simulink model "Sliding_Mode_Slotine_Regressor"  (R2018b)
settings: Solver=FixedStepAuto  StartTime=0.0  StopTime=10  FixedStep=0.001  RelTol=1e-3
values from neighbouring files (symbols this model uses):
  F1G = 0.2    [Main_Code.m]    (also in Main_Code_Gravity_Compensation.m)
  F2G = 0.2    [Main_Code.m]    (also in Main_Code_Gravity_Compensation.m)
  F3G = 0.005    [Main_Code.m]    (also in Main_Code_Gravity_Compensation.m)
  Gauss_B = [0 0 0 0 0 0 0 0 0 0 0 0 ... (1200 elements, 15x80)]    [Gauss_Jordan.mat]
  Gauss_BB = [0 0 0 0 0 0 0 0 0 0 0 0 ... (1200 elements, 80x15)]    [Gauss_Jordan.mat]
  phi_Dynamic = [phi0;phi1;phi2;phi3;phi4;phi5;phi6;phi7]    [Parameters_Builder.m]    (also in Robot_Parameters.mat = [0.73163251 -0.0393 0 2.40643096032e-18 0.000785329049449 0.; Robot_Parameters_Ident.mat = [0.78122 -0.0393 0 2.40643096032e-18 0.000785329049449 0.000; Robot_Parameters_Ident_With_Disturbance.mat = [0.78122 -0.0393 0 2.40643096032e-18 0.000785329049449 0.000)
  phi_Kinematic = [l__0;l__1;l__3;l__5;l__2;l__7;theta;alpha;d__0;l__x35;l__z35;psi0]    [Parameters_Builder.m]    (also in Robot_Parameters.mat = [0.006 0.182 0.05 0.115 0.07 0.0342 0.733038285838 0.8726646; Robot_Parameters_Ident.mat = [0.006 0.182 0.05 0.115 0.07 0.0342 0.733038285838 0.8726646; Robot_Parameters_Ident_With_Disturbance.mat = [0.006 0.182 0.05 0.115 0.07 0.0342 0.733038285838 0.8726646)
undefined symbols (not defined in the file or in its folder): gamma, K
libraries: slrtlib x5, xpcrtudplib x3, xpcutilitieslib x2
settings Model: Creator=Legend  LastModifiedBy=ARAS
settings SFSimCC: SimUseLocalCustomCode=off
settings RTWCC: RTWUseLocalCustomCode=off
settings CodeAppCC: StateflowObjectComments=on

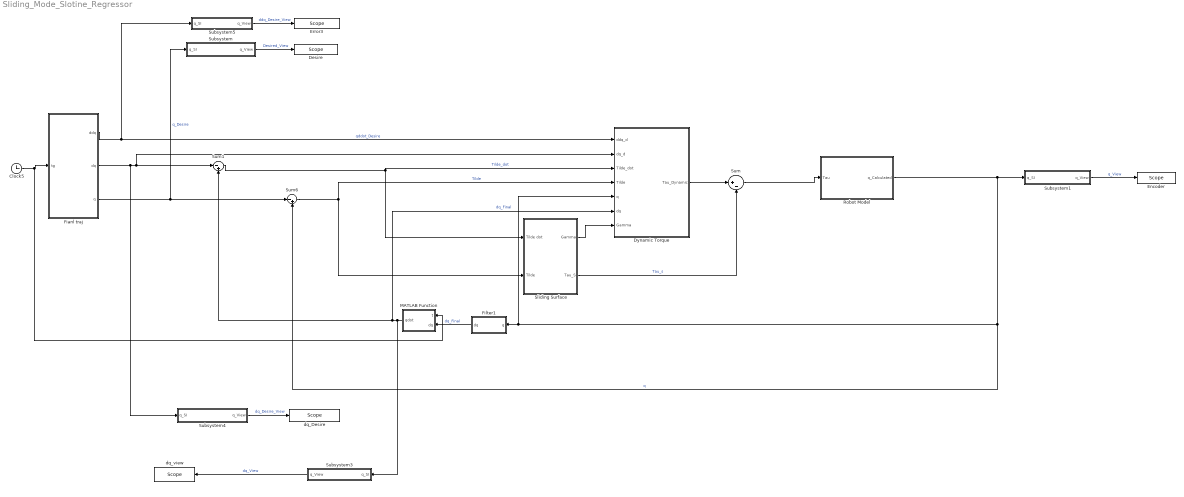
== system Sliding_Mode_Slotine_Regressor ==
  Clock5 : Clock
  Desire : slrtlib/Displays and Logging/Scope   scopeno=2  scopetype=Target  autostart=on  viewmode=Numerical  formatstr='%15.6f'  grid=on  ylimits=[0,0]  nosamples=3  noprepostsamples=0  interleave=1  triggermode=FreeRun  triggersignal=1  trigsignalfromport=off  triggerlevel=0.0  triggerslope=Either  triggerscope=1  triggersample=0  filename=data.dat  mode=Lazy  writesize=512  autorestart=off  dynamicfilemode=off  maxwritefilesize=512*1024^2
  Dynamic Torque : Subsystem
  Encoder : slrtlib/Displays and Logging/Scope   scopeno=1  scopetype=Target  autostart=on  viewmode=Numerical  formatstr='%15.6f'  grid=on  ylimits=[0,0]  nosamples=3  noprepostsamples=0  interleave=1  triggermode=FreeRun  triggersignal=1  trigsignalfromport=off  triggerlevel=0.0  triggerslope=Either  triggerscope=1  triggersample=0  filename=data.dat  mode=Lazy  writesize=512  autorestart=off  dynamicfilemode=off  maxwritefilesize=512*1024^2
  Error3 : slrtlib/Displays and Logging/Scope   scopeno=3  scopetype=Target  autostart=on  viewmode=Numerical  formatstr='%15.6f'  grid=on  ylimits=[0,0]  nosamples=3  noprepostsamples=0  interleave=1  triggermode=FreeRun  triggersignal=1  trigsignalfromport=off  triggerlevel=0.0  triggerslope=Either  triggerscope=1  triggersample=0  filename=data.dat  mode=Lazy  writesize=512  autorestart=off  dynamicfilemode=off  maxwritefilesize=512*1024^2
  Fianl traj : MATLAB Function  TreatAsAtomicUnit=on
  Filter1 : Subsystem
  MATLAB Function : MATLAB Function  TreatAsAtomicUnit=on
  Robot Model : Subsystem
  Sliding Surface : Subsystem
  Subsystem : Subsystem
  Subsystem1 : Subsystem
  Subsystem3 : Subsystem
  Subsystem4 : Subsystem
  Subsystem5 : Subsystem
  Sum : Sum  Inputs=|+-
  Sum1 : Sum  Inputs=|-+
  Sum6 : Sum  Inputs=|-+
  dq_Desire : slrtlib/Displays and Logging/Scope   scopeno=4  scopetype=Target  autostart=on  viewmode=Numerical  formatstr='%15.6f'  grid=on  ylimits=[0,0]  nosamples=3  noprepostsamples=0  interleave=1  triggermode=FreeRun  triggersignal=1  trigsignalfromport=off  triggerlevel=0.0  triggerslope=Either  triggerscope=1  triggersample=0  filename=data.dat  mode=Lazy  writesize=512  autorestart=off  dynamicfilemode=off  maxwritefilesize=512*1024^2
  dq_view : slrtlib/Displays and Logging/Scope   scopeno=5  scopetype=Target  autostart=on  viewmode=Numerical  formatstr='%15.6f'  grid=on  ylimits=[0,0]  nosamples=3  noprepostsamples=0  interleave=1  triggermode=FreeRun  triggersignal=1  trigsignalfromport=off  triggerlevel=0.0  triggerslope=Either  triggerscope=1  triggersample=0  filename=data.dat  mode=Lazy  writesize=512  autorestart=off  dynamicfilemode=off  maxwritefilesize=512*1024^2
  wires:
  MATLAB Function/1(qdot) -> Sum1/2, Dynamic Torque/6(dq), Subsystem3/1(q_SI)  "dq_Final"
  Robot Model/1(q_Calculated) -> Subsystem1/1(q_SI), Dynamic Torque/5(q), Filter1/1(q), Sum6/2  "q"
  Clock5/1 -> MATLAB Function/1(t), Fianl traj/1(tg)
  Sum6/1 -> Dynamic Torque/4(Tilde), Sliding Surface/2(Tilde)  "Tilde"
  Sum1/1 -> Sliding Surface/1(Tilde dot), Dynamic Torque/3(Tilde_dot)  "Tilde_dot"
  Fianl traj/1(ddq) -> Subsystem5/1(q_SI), Dynamic Torque/1(ddq_d)  "qddot_Desire"
  Sum/1 -> Robot Model/1(Tau)
  Dynamic Torque/1(Tau_Dynamic) -> Sum/1
  Sliding Surface/2(Tau_S) -> Sum/2  "Tau_s"
  Sliding Surface/1(Gamma) -> Dynamic Torque/7(Gamma)
  Subsystem1/1(q_View) -> Encoder/1  "q_View"
  Fianl traj/3(q) -> Subsystem/1(q_SI), Sum6/1  "q_Desire"
  Fianl traj/2(dq) -> Dynamic Torque/2(dq_d), Sum1/1, Subsystem4/1(q_SI)
  Subsystem5/1(q_View) -> Error3/1  "ddq_Desire_View"
  Subsystem/1(q_View) -> Desire/1  "Desired_View"
  Subsystem4/1(q_View) -> dq_Desire/1  "dq_Desire_View"
  Filter1/1(dq) -> MATLAB Function/2(dq)  "dq_Final"
  Subsystem3/1(q_View) -> dq_view/1  "dq_View"

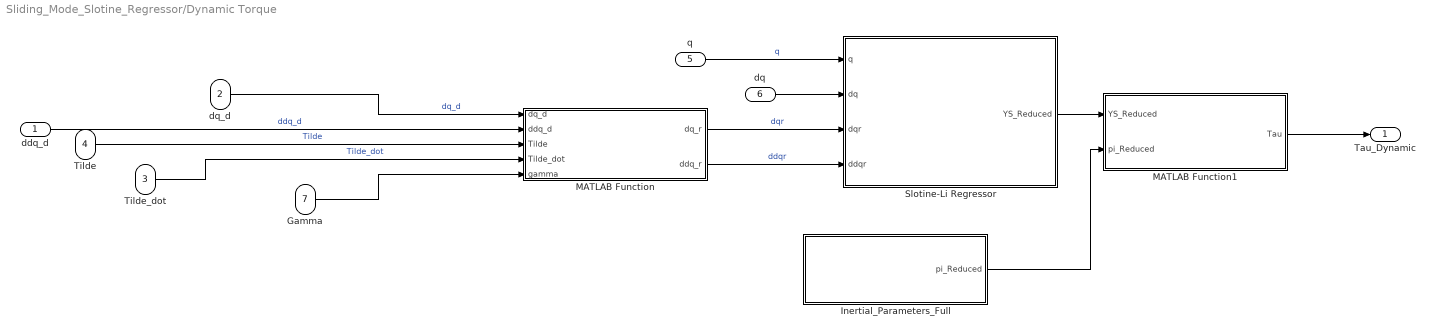
== system Sliding_Mode_Slotine_Regressor/Dynamic Torque ==
  ddq_d : Inport
  dq_d : Inport  Port=2
  Tilde_dot : Inport  Port=3
  Tilde : Inport  Port=4
  q : Inport  Port=5
  dq : Inport  Port=6
  Gamma : Inport  Port=7
  Inertial_Parameters_Full : Subsystem
  MATLAB Function : MATLAB Function  TreatAsAtomicUnit=on
  MATLAB Function1 : MATLAB Function  TreatAsAtomicUnit=on
  Slotine-Li Regressor : Subsystem
  Tau_Dynamic : Outport
  wires:
  MATLAB Function1/1(Tau) -> Tau_Dynamic/1
  dq_d/1 -> MATLAB Function/1(dq_d)  "dq_d"
  Tilde_dot/1 -> MATLAB Function/4(Tilde_dot)  "Tilde_dot"
  Tilde/1 -> MATLAB Function/3(Tilde)  "Tilde"
  ddq_d/1 -> MATLAB Function/2(ddq_d)  "ddq_d"
  Gamma/1 -> MATLAB Function/5(gamma)
  q/1 -> Slotine-Li Regressor/1(q)  "q"
  dq/1 -> Slotine-Li Regressor/2(dq)
  MATLAB Function/1(dq_r) -> Slotine-Li Regressor/3(dqr)  "dqr"
  MATLAB Function/2(ddq_r) -> Slotine-Li Regressor/4(ddqr)  "ddqr"
  Slotine-Li Regressor/1(YS_Reduced) -> MATLAB Function1/1(YS_Reduced)
  Inertial_Parameters_Full/1("pi_Reduced ") -> MATLAB Function1/2(pi_Reduced)

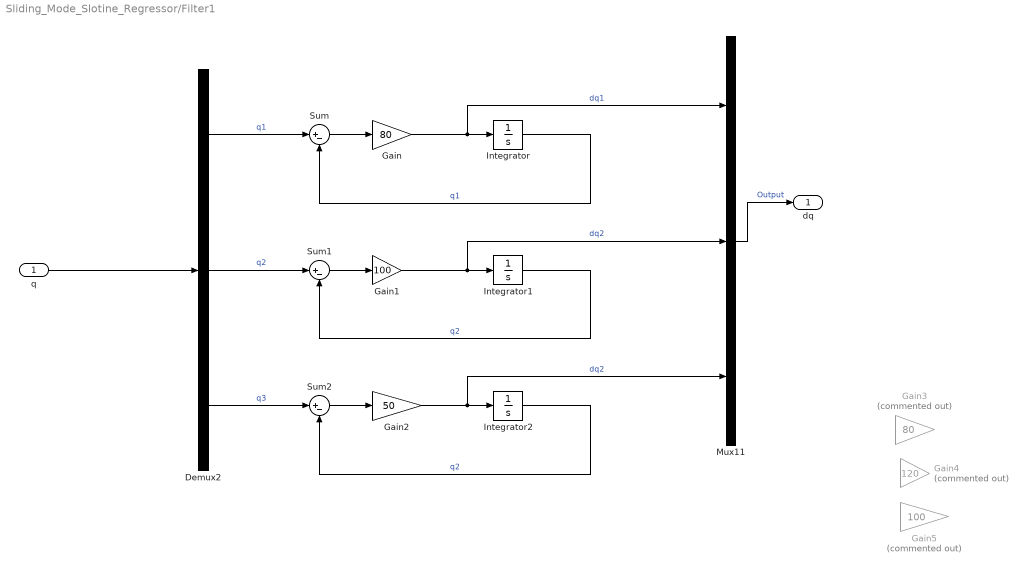
== system Sliding_Mode_Slotine_Regressor/Filter1 ==
  q : Inport
  Demux2 : Demux  Outputs=3
  Gain : Gain  Gain=80
  Gain1 : Gain  Gain=100
  Gain2 : Gain  Gain=50
  Gain3 : Gain  Commented=on  Gain=80
  Gain4 : Gain  Commented=on  Gain=120
  Gain5 : Gain  Commented=on  Gain=100
  Integrator : Integrator
  Integrator1 : Integrator
  Integrator2 : Integrator
  Mux11 : Mux  Inputs=3
  Sum : Sum  Inputs=|+-
  Sum1 : Sum  Inputs=|+-
  Sum2 : Sum  Inputs=|+-
  dq : Outport
  wires:
  Mux11/1 -> dq/1  "Output"
  q/1 -> Demux2/1
  Demux2/1 -> Sum/1  "q1"
  Sum/1 -> Gain/1
  Integrator/1 -> Sum/2  "q1"
  Gain/1 -> Mux11/1, Integrator/1  "dq1"
  Gain1/1 -> Mux11/2, Integrator1/1  "dq2"
  Demux2/2 -> Sum1/1  "q2"
  Sum1/1 -> Gain1/1
  Integrator1/1 -> Sum1/2  "q2"
  Integrator2/1 -> Sum2/2  "q2"
  Demux2/3 -> Sum2/1  "q3"
  Sum2/1 -> Gain2/1
  Gain2/1 -> Mux11/3, Integrator2/1  "dq2"

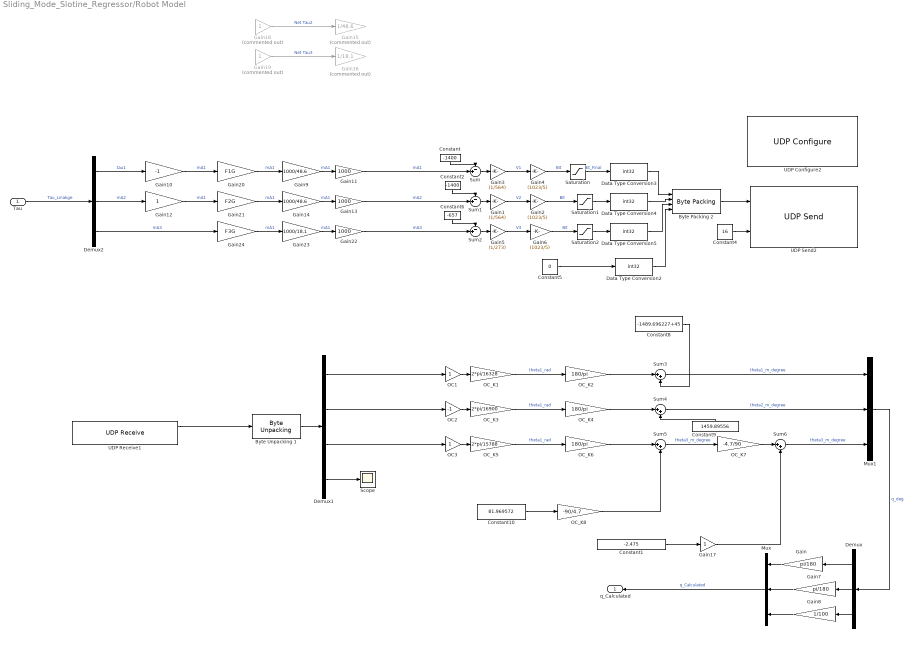
== system Sliding_Mode_Slotine_Regressor/Robot Model ==
  Tau : Inport
  Byte Packing 2 : xpcutilitieslib/Byte Packing   MaskPackedDataType=uint8  MaskUnpackedDataTypes={'int32','int32','int32','int32'}  MaskAlignment=1
  Byte Unpacking 1 : xpcutilitieslib/Byte Unpacking   MaskUnpackedDataTypes={'int32'}  MaskUnpackedDataSizes={[4]}  MaskAlignment=1
      settings: SourceProductName=Simulink Real-Time  SourceProductBaseCode=XP
  Constant : Constant  Value=-1400
  Constant1 : Constant  Value=-2.475
  Constant10 : Constant  Value=81.969572
  Constant2 : Constant  Value=-1400
  Constant4 : Constant  Value=16
  Constant5 : Constant  Value=0
  Constant6 : Constant  Value=-657
  Constant8 : Constant  Value=-1489.696227+45
  Constant9 : Constant  Value=1459.89556
  Data Type Conversion{2..5} (4 alike) : DataTypeConversion  OutDataTypeStr=int32
  Demux : Demux  Outputs=3
  Demux1 : Demux
  Demux2 : Demux  Outputs=3
  Gain : Gain  Gain=pi/180
  Gain1 : Gain  Gain=(1/564)
  Gain10 : Gain  Gain=-1
  Gain11 : Gain  Gain=1000
  Gain12 : Gain
  Gain13 : Gain  Gain=1000
  Gain14 : Gain  Gain=1000/48.6
  Gain15 : Gain  Commented=on  Gain=1/48.6
  Gain16 : Gain  Commented=on  Gain=1/18.1
  Gain17 : Gain
  Gain18 : Gain  Commented=on
  Gain19 : Gain  Commented=on
  Gain2 : Gain  Gain=(1023/5)
  Gain20 : Gain  Gain=F1G
  Gain21 : Gain  Gain=F2G
  Gain22 : Gain  Gain=1000
  Gain23 : Gain  Gain=1000/18.1
  Gain24 : Gain  Gain=F3G
  Gain3 : Gain  Gain=(1/564)
  Gain4 : Gain  Gain=(1023/5)
  Gain5 : Gain  Gain=(1/273)
  Gain6 : Gain  Gain=(1023/5)
  Gain7 : Gain  Gain=pi/180
  Gain8 : Gain  Gain=1/100
  Gain9 : Gain  Gain=1000/48.6
  Mux : Mux  Inputs=3
  Mux1 : Mux  Inputs=3
  OC1 : Gain  ParamDataTypeStr=double  OutDataTypeStr=double
  OC2 : Gain  Gain=-1  ParamDataTypeStr=double  OutDataTypeStr=double
  OC3 : Gain  ParamDataTypeStr=double  OutDataTypeStr=double
  OC_K1 : Gain  Gain=2*pi/16328  ParamDataTypeStr=double  OutDataTypeStr=double
  OC_K2 : Gain  Gain=180/pi  ParamDataTypeStr=double  OutDataTypeStr=double
  OC_K3 : Gain  Gain=2*pi/16900  ParamDataTypeStr=double  OutDataTypeStr=double
  OC_K4 : Gain  Gain=180/pi  ParamDataTypeStr=double  OutDataTypeStr=double
  OC_K5 : Gain  Gain=2*pi/15788  ParamDataTypeStr=double  OutDataTypeStr=double
  OC_K6 : Gain  Gain=180/pi  ParamDataTypeStr=double  OutDataTypeStr=double
  OC_K7 : Gain  Gain=-4.7/90  ParamDataTypeStr=double  OutDataTypeStr=double
  OC_K8 : Gain  Gain=-90/4.7  ParamDataTypeStr=double  OutDataTypeStr=double
  Saturation : Saturate  UpperLimit=1023  LowerLimit=0
  Saturation1 : Saturate  UpperLimit=1023  LowerLimit=0
  Saturation2 : Saturate  UpperLimit=1023  LowerLimit=0
  Scope : Scope
  Sum : Sum  Inputs=-+|
  Sum1 : Sum  Inputs=-+|
  Sum2 : Sum  Inputs=-+|
  Sum{3..6} (4 alike) : Sum  Inputs=|++
  UDP Configure2 : xpcrtudplib/UDP Configure  Priority=-1  IpAddress=192.168.1.4  SubnetMask=255.255.255.0  Gateway=0.0.0.0  PciBus=[3]  PciSlot=[1]  PciFunction=0  ID=1  tune=0  disable=off  enableMulticast=off  MulticastIpAddress={}  MulticastMask={}
      settings: SourceProductName=Simulink Real-Time  SourceProductBaseCode=XP
  UDP Receive1 : xpcrtudplib/UDP Receive  ipAddressVal=192.168.1.4  localPort=5500  rcvWidth=16  rcvFmAny=on  fmAddress=0.0.0.0  rcvMulticast=off  multicastAddress={}  maxUDPQueue=8  sampleTime=0.001
      settings: SourceProductName=Simulink Real-Time
  UDP Send2 : xpcrtudplib/UDP Send  ipAddressVal=192.168.1.4  localPort=5500  toAddress=192.168.1.3  toPort=5500  sampleTime=0.001
      settings: SourceProductName=Simulink Real-Time  SourceProductBaseCode=XP
  q_Calculated : Outport
  wires:
  Demux1/2 -> OC2/1
  Sum/1 -> Gain3/1
  Data Type Conversion2/1 -> Byte Packing 2/4
  OC_K1/1 -> OC_K2/1  "theta1_rad"
  Byte Packing 2/1 -> UDP Send2/1
  Gain4/1 -> Saturation/1  "Bit"
  OC1/1 -> OC_K1/1
  Constant4/1 -> UDP Send2/2
  UDP Receive1/1 -> Byte Unpacking 1/1
  OC_K2/1 -> Sum3/1
  Data Type Conversion3/1 -> Byte Packing 2/1
  Data Type Conversion4/1 -> Byte Packing 2/2
  Data Type Conversion5/1 -> Byte Packing 2/3
  Demux1/3 -> OC3/1
  Constant5/1 -> Data Type Conversion2/1
  OC_K4/1 -> Sum4/1
  Constant/1 -> Sum/1
  Saturation/1 -> Data Type Conversion3/1  "Bit_Final"
  Constant10/1 -> OC_K8/1
  Gain3/1 -> Gain4/1  "V1"
  OC_K6/1 -> Sum5/1
  Saturation2/1 -> Data Type Conversion5/1
  Constant6/1 -> Sum2/1
  Gain6/1 -> Saturation2/1  "Bit"
  Gain5/1 -> Gain6/1  "V3"
  Sum2/1 -> Gain5/1
  Byte Unpacking 1/1 -> Demux1/1
  Sum1/1 -> Gain1/1
  Sum4/1 -> Mux1/2  "theta2_m_degree"
  Demux1/1 -> OC1/1
  Mux1/1 -> Demux/1  "q_deg"
  OC_K3/1 -> OC_K4/1  "theta1_rad"
  OC_K5/1 -> OC_K6/1  "theta1_rad"
  OC3/1 -> OC_K5/1
  Gain2/1 -> Saturation1/1  "Bit"
  Demux/1 -> Gain/1
  Tau/1 -> Demux2/1  "Tau_Linakge"
  Gain/1 -> Mux/1
  OC2/1 -> OC_K3/1
  Sum3/1 -> Mux1/1  "theta1_m_degree"
  Demux1/4 -> Scope/1
  Demux/2 -> Gain7/1
  Gain1/1 -> Gain2/1  "V2"
  Gain7/1 -> Mux/2
  Constant8/1 -> Sum3/2
  Constant9/1 -> Sum4/2
  Constant2/1 -> Sum1/1
  Saturation1/1 -> Data Type Conversion4/1
  Mux/1 -> q_Calculated/1  "q_Calculated"
  Gain18/1 -> Gain15/1  "Net Tau2"
  Gain19/1 -> Gain16/1  "Net Tau3"
  Demux2/1 -> Gain10/1  "tau1"
  Gain9/1 -> Gain11/1  "mA1"
  Gain10/1 -> Gain20/1  "mA1"
  Gain11/1 -> Sum/2  "mA1"
  Gain14/1 -> Gain13/1  "mA1"
  Gain12/1 -> Gain21/1  "mA1"
  Gain13/1 -> Sum1/2  "mA2"
  Demux2/2 -> Gain12/1  "mA2"
  Demux/3 -> Gain8/1
  Gain8/1 -> Mux/3
  Gain23/1 -> Gain22/1  "mA1"
  Gain22/1 -> Sum2/2  "mA3"
  Demux2/3 -> Gain24/1  "mA3"
  OC_K8/1 -> Sum5/2
  Sum5/1 -> OC_K7/1  "theta3_m_degree"
  OC_K7/1 -> Sum6/1
  Sum6/1 -> Mux1/3  "theta3_m_degree"
  Constant1/1 -> Gain17/1
  Gain17/1 -> Sum6/2
  Gain20/1 -> Gain9/1  "mA1"
  Gain21/1 -> Gain14/1  "mA1"
  Gain24/1 -> Gain23/1  "mA1"

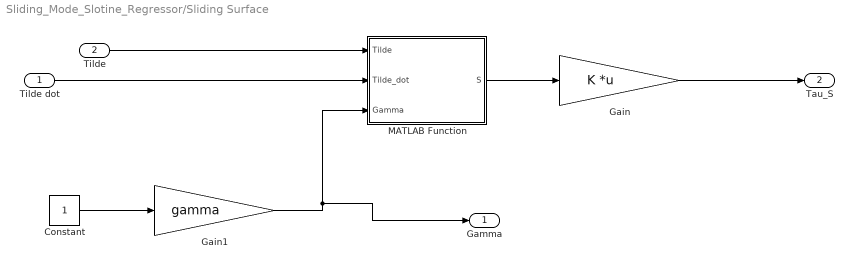
== system Sliding_Mode_Slotine_Regressor/Sliding Surface ==
  Tilde dot : Inport
  Tilde : Inport  Port=2
  Constant : Constant
  Gain : Gain  Gain=K  Multiplication=Matrix(K*u)
  Gain1 : Gain  Gain=gamma
  MATLAB Function : MATLAB Function  TreatAsAtomicUnit=on
  Gamma : Outport
  Tau_S : Outport  Port=2
  wires:
  Tilde dot/1 -> MATLAB Function/2(Tilde_dot)
  MATLAB Function/1(S) -> Gain/1
  Tilde/1 -> MATLAB Function/1(Tilde)
  Gain/1 -> Tau_S/1
  Constant/1 -> Gain1/1
  Gain1/1 -> Gamma/1, MATLAB Function/3(Gamma)

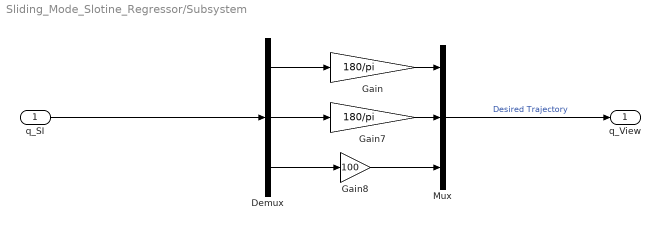
== system Sliding_Mode_Slotine_Regressor/Subsystem ==
  q_SI : Inport
  Demux : Demux  Outputs=3
  Gain : Gain  Gain=180/pi
  Gain7 : Gain  Gain=180/pi
  Gain8 : Gain  Gain=100
  Mux : Mux  Inputs=3
  q_View : Outport
  wires:
  Gain7/1 -> Mux/2
  Demux/3 -> Gain8/1
  Gain8/1 -> Mux/3
  Demux/2 -> Gain7/1
  q_SI/1 -> Demux/1
  Gain/1 -> Mux/1
  Demux/1 -> Gain/1
  Mux/1 -> q_View/1  "Desired Trajectory"

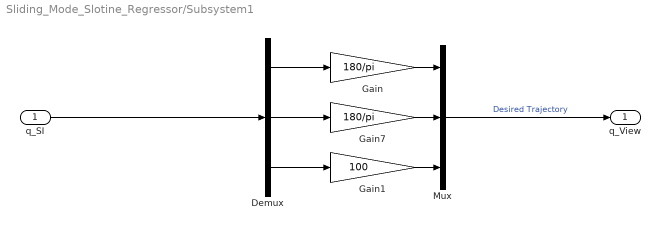
== system Sliding_Mode_Slotine_Regressor/Subsystem1 ==
  q_SI : Inport
  Demux : Demux  Outputs=3
  Gain : Gain  Gain=180/pi
  Gain1 : Gain  Gain=100
  Gain7 : Gain  Gain=180/pi
  Mux : Mux  Inputs=3
  q_View : Outport
  wires:
  Gain7/1 -> Mux/2
  Demux/3 -> Gain1/1
  Demux/2 -> Gain7/1
  q_SI/1 -> Demux/1
  Gain/1 -> Mux/1
  Demux/1 -> Gain/1
  Mux/1 -> q_View/1  "Desired Trajectory"
  Gain1/1 -> Mux/3

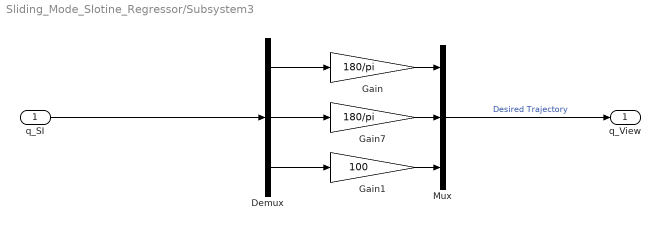
== system Sliding_Mode_Slotine_Regressor/Subsystem3 ==
  q_SI : Inport
  Demux : Demux  Outputs=3
  Gain : Gain  Gain=180/pi
  Gain1 : Gain  Gain=100
  Gain7 : Gain  Gain=180/pi
  Mux : Mux  Inputs=3
  q_View : Outport
  wires:
  Gain7/1 -> Mux/2
  Demux/3 -> Gain1/1
  Demux/2 -> Gain7/1
  q_SI/1 -> Demux/1
  Gain/1 -> Mux/1
  Demux/1 -> Gain/1
  Mux/1 -> q_View/1  "Desired Trajectory"
  Gain1/1 -> Mux/3

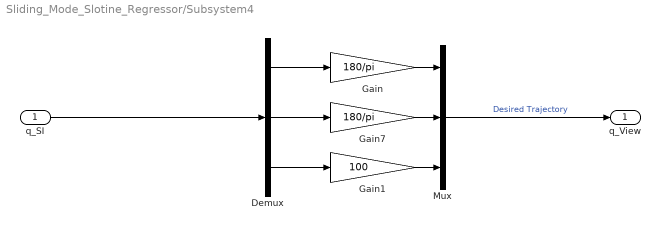
== system Sliding_Mode_Slotine_Regressor/Subsystem4 ==
  q_SI : Inport
  Demux : Demux  Outputs=3
  Gain : Gain  Gain=180/pi
  Gain1 : Gain  Gain=100
  Gain7 : Gain  Gain=180/pi
  Mux : Mux  Inputs=3
  q_View : Outport
  wires:
  Gain7/1 -> Mux/2
  Demux/3 -> Gain1/1
  Demux/2 -> Gain7/1
  q_SI/1 -> Demux/1
  Gain/1 -> Mux/1
  Demux/1 -> Gain/1
  Mux/1 -> q_View/1  "Desired Trajectory"
  Gain1/1 -> Mux/3

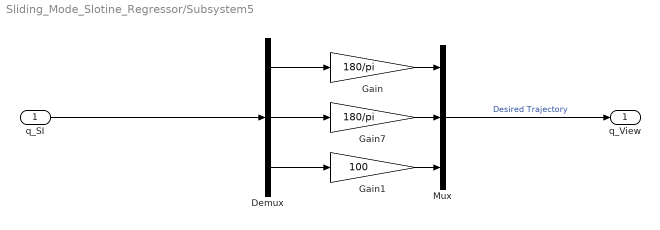
== system Sliding_Mode_Slotine_Regressor/Subsystem5 ==
  q_SI : Inport
  Demux : Demux  Outputs=3
  Gain : Gain  Gain=180/pi
  Gain1 : Gain  Gain=100
  Gain7 : Gain  Gain=180/pi
  Mux : Mux  Inputs=3
  q_View : Outport
  wires:
  Gain7/1 -> Mux/2
  Demux/3 -> Gain1/1
  Demux/2 -> Gain7/1
  q_SI/1 -> Demux/1
  Gain/1 -> Mux/1
  Demux/1 -> Gain/1
  Mux/1 -> q_View/1  "Desired Trajectory"
  Gain1/1 -> Mux/3

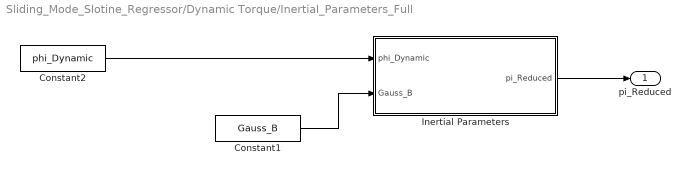
== system Sliding_Mode_Slotine_Regressor/Dynamic Torque/Inertial_Parameters_Full ==
  Constant1 : Constant  Value=Gauss_B
  Constant2 : Constant  Value=phi_Dynamic
  Inertial Parameters : MATLAB Function  TreatAsAtomicUnit=on
  "pi_Reduced " : Outport
  wires:
  Inertial Parameters/1(pi_Reduced) -> "pi_Reduced "/1
  Constant2/1 -> Inertial Parameters/1(phi_Dynamic)
  Constant1/1 -> Inertial Parameters/2(Gauss_B)

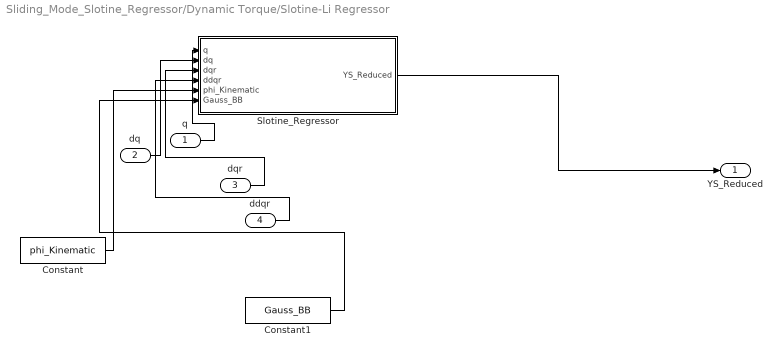
== system Sliding_Mode_Slotine_Regressor/Dynamic Torque/Slotine-Li Regressor ==
  q : Inport
  dq : Inport  Port=2
  dqr : Inport  Port=3
  ddqr : Inport  Port=4
  Constant : Constant  Value=phi_Kinematic
  Constant1 : Constant  Value=Gauss_BB
  Slotine_Regressor : MATLAB Function  TreatAsAtomicUnit=on
  YS_Reduced : Outport
  wires:
  Slotine_Regressor/1(YS_Reduced) -> YS_Reduced/1
  Constant/1 -> Slotine_Regressor/5(phi_Kinematic)
  q/1 -> Slotine_Regressor/1(q)
  dq/1 -> Slotine_Regressor/2(dq)
  dqr/1 -> Slotine_Regressor/3(dqr)
  ddqr/1 -> Slotine_Regressor/4(ddqr)
  Constant1/1 -> Slotine_Regressor/6(Gauss_BB)

== matlab function Sliding_Mode_Slotine_Regressor/Dynamic Torque/MATLAB Function1 ==
  data: Tau output; YS_Reduced input; pi_Reduced input
function Tau  = fcn(YS_Reduced,pi_Reduced)

Tau=YS_Reduced*pi_Reduced;

end

== matlab function Sliding_Mode_Slotine_Regressor/Sliding Surface/MATLAB Function ==
  data: Tilde input; S output; Tilde_dot input; Gamma input
function S = fcn(Tilde,Tilde_dot,Gamma)

S=Tilde_dot+Gamma*Tilde;

%Tau_S=-K*S;

end

== matlab function Sliding_Mode_Slotine_Regressor/MATLAB Function ==
  data: t input; qdot output; dq input
function qdot = fcn(t,dq)

if t<0.5
    
    qdot=[0;0;0];
    
    
else qdot=dq;
    
end



end

== matlab function Sliding_Mode_Slotine_Regressor/Dynamic Torque/Inertial_Parameters_Full/Inertial Parameters ==
  data: pi_Reduced output; phi_Dynamic input; Gauss_B input
function pi_Reduced  = fcn(phi_Dynamic,Gauss_B)

pi_Full= Inertial_Parameters_Full(phi_Dynamic);
pi_Reduced=Gauss_B*pi_Full;

end

== matlab function Sliding_Mode_Slotine_Regressor/Dynamic Torque/Slotine-Li Regressor/Slotine_Regressor ==
  data: q input; dq input; dqr input; ddqr input; YS_Reduced output; phi_Kinematic input; Gauss_BB input
function YS_Reduced = fcn(q,dq,dqr,ddqr,phi_Kinematic,Gauss_BB)

YS_Full = Slotine_Regressor(q,dq,dqr,ddqr,phi_Kinematic);
YS_Reduced=YS_Full*Gauss_BB;

end

== matlab function Sliding_Mode_Slotine_Regressor/Dynamic Torque/MATLAB Function ==
  data: dq_r output; ddq_r output; dq_d input; ddq_d input; Tilde input; Tilde_dot input; gamma input
function [dq_r,ddq_r] = fcn(dq_d,ddq_d,Tilde,Tilde_dot,gamma)

dq_r=dq_d-gamma*Tilde;
ddq_r=ddq_d-gamma*Tilde_dot;

end

== matlab function Sliding_Mode_Slotine_Regressor/Fianl traj ==
  settings: updateMethod=DISCRETE
  data: ddq output; dq output; q output; tg input
function [ddq,dq,q]   = fcn(tg)

a=0.5;

t=tg;

%% Trajectory Define

Aq1=42.5;
Aq2=41.5;
Aq3=-1.8;


    q1=Aq1*sin(a*t);
    q2=Aq2*cos(a*t)+18.5;
    q3=Aq3*sin(a*t)-0.4;
    q=[q1*(pi/180);q2*(pi/180);q3/100];

    dq1=+a*Aq1*cos(a*t);
    dq2=-a*Aq2*sin(a*t);
    dq3=+a*Aq3*cos(a*t);
    dq=[dq1*(pi/180);dq2*(pi/180);dq3/100];

    ddq1=-a*a*Aq1*sin(a*t);
    ddq2=-a*a*Aq2*cos(a*t);
    ddq3=-a*a*Aq3*sin(a*t);
    ddq=[ddq1*(pi/180);ddq2*(pi/180);ddq3/100];





end
